simulink model "lift_stateflow"  (R2020b)
settings: Solver=VariableStepAuto  StartTime=0.0  StopTime=10.0  RelTol=1e-3
settings Model: Creator=shraddha  LastModifiedBy=shraddha

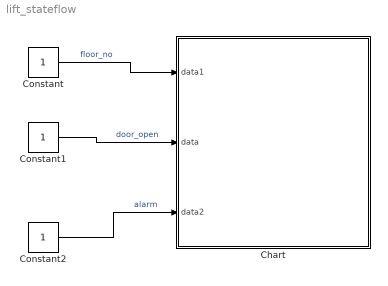
== system lift_stateflow ==
  Chart : Stateflow chart  TreatAsAtomicUnit=on
  Constant : Constant
  Constant1 : Constant
  Constant2 : Constant
  wires:
  Constant1/1 -> Chart/2(data)  "door_open"
  Constant/1 -> Chart/1(data1)  "floor_no"
  Constant2/1 -> Chart/3(data2)  "alarm"

== stateflow chart lift_stateflow/Chart ==
  state LIFT_A
    state OPERATION [parallel]
      settings: executionOrder=1
      state floor0
      state floor4
      state floor1
      state floor3
      state floor2
      (default) -> floor0
      floor0 -> floor0 [order 2] : [door_open~=0]
      floor4 -> floor4 [order 2] : [door_open~=0]
      floor0 -> floor1 [order 1] : [floor_no>0]
      floor1 -> floor0 [order 2] : [floor_no<1]
      floor4 -> floor3 [order 1] : [floor_no<4]
      floor3 -> floor4 [order 1] : [floor_no>3]
      floor1 -> floor1 [order 3] : [door_open~=0]
      floor3 -> floor3 [order 3] : [door_open~=0]
      floor1 -> floor2 [order 1] : [floor_no>1]
      floor2 -> floor1 [order 2] : [floor_no<2]
      floor2 -> floor3 [order 1] : [floor_no>2]
      floor3 -> floor2 [order 2] : [floor_no<3]
      floor2 -> floor2 [order 3] : [door_open~=0]
    state ALARM [parallel]
      settings: executionOrder=2
      state ON
      state OFF
      ON -> OFF : [alarm~=1]
      OFF -> ON : [alarm~=0]
      (default) -> OFF
  (default) -> LIFT_A
  data: data1 input; data input; data2 input
